simulink library "sm_mining_loader_lib"  (R2026a)
settings: Solver=VariableStepAuto
undefined symbols (not defined in the file): FL, FR, Init, LL, LR, Maneuver, minMachParams, motGradParams, RL, RR, simscape, SL, SR, T, X, Y, Z
libraries: sm_lib x130, nesl_utility x77, fl_lib x36, sdl_lib x11, simulink x4, $bdroot x3, sm_vehicle_utilities_lib x2, simulink_extras x2, statsLibrary x1, grid_element x1, Maneuver_Get_Pose x1
(part 1 of 6)
settings Model: Creator=smiller  LastModifiedBy=smiller

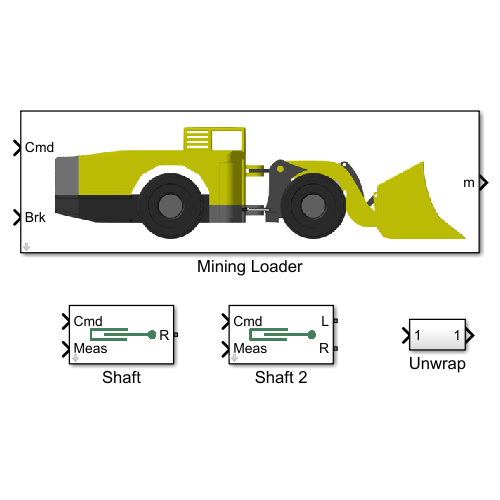
[thumbnail: Simulink's stored preview of the top-level diagram]
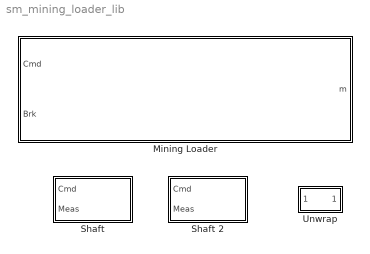
== system sm_mining_loader_lib ==
  Mining Loader : Subsystem  mask{popup_steer_actuation=Hinge Motion, popup_lift_actuation=Hinge Motion, popup_tilt_actuation=Hinge Motion, popup_scene=Grid, popup_sensor=None}
      mask prompts: popup_steer_actuation "Steer Actuation"; popup_lift_actuation "Lift Actuation"; popup_tilt_actuation "Tilt Actuation"; popup_scene "Scene"; popup_sensor "Sensor"
      mask init:
      | bh = gcb;
      | 
      | liftAct = get_param(bh,'popup_lift_actuation');
      | tiltAct = get_param(bh,'popup_tilt_actuation');
      | steerAct = get_param(bh,'popup_steer_actuation');
      | 
      | if(strcmp(liftAct,'Cylinder Actuation'))
      |     liftActStr = 'Shaft';
      | else
      |     liftActStr = 'Position';
      | end
      | if(strcmp(tiltAct,'Cylinder Actuation'))
      |     tiltActStr = 'Shaft';
      | else
      |     tiltActStr = 'Position';
      | end
      | if(strcmp(steerAct,'Cylinder Actuation'))
      |     steerActStr = 'Shaft';
      | else
      |     steerActStr = 'Position';
      | end
      | 
      | set_param([bh '/Actuation'],...
      |     'popup_lift_actuation',liftActStr,...
      |     'popup_tilt_actuation',tiltActStr,...
      |     'popup_steer_actuation',steerActStr...
      |     );
      | 
      | set_param([bh '/Scene'],...
      |     'LabelModeActiveChoice',get_param(bh,'popup_scene'))
      mask TypeOptions popup_steer_actuation: Vehicle/popup_steer_actuation
      mask TypeOptions popup_lift_actuation: Vehicle/popup_lift_actuation
      mask TypeOptions popup_tilt_actuation: Vehicle/popup_tilt_actuation
      mask TypeOptions popup_scene: SlopeX | Grid
      mask TypeOptions popup_sensor: Braking Distance Sensor/popup_sensor
      mask Display: image('sm_mining_loader_IMAGE.png')
  Shaft : Subsystem  VariantControl=Shaft  mask{Kp=motGradParams.bladeTilt.propGain, Ki=motGradParams.bladeTilt.integral, Kd=motGradParams.bladeTilt.derivative, p_init=motGradParams.bladeTilt.initPos, f_init=-4.07e4*3}
      mask prompts: Kp "Proportional Gain"; Ki "Integral Gain"; Kd "Derivative Gain"; p_init "Initial Position"; f_init "Initial Force"
      mask Display: image('sm_mining_loader_actuation_Shaft_IMAGE.png')
  Shaft 2 : Subsystem  VariantControl=Shaft  mask{Kp=minMachParams.Control.Steer.propGain, Ki=minMachParams.Control.Steer.intgGain, Kd=minMachParams.Control.Steer.dervGain, p_init=minMachParams.Control.Steer.initPos, popup_act_pair=Parallel}
      mask prompts: Kp "Proportional Gain"; Ki "Integral Gain"; Kd "Derivative Gain"; p_init "Initial Position"; popup_act_pair "Actuator Pair"
      mask init:
      | bh = gcb;
      | pairMode = get_param(bh,'popup_act_pair');
      | if(strcmp(pairMode,'Parallel'))
      | set_param([bh '/Sign L'],'Gain','1')
      | else
      |     set_param([bh '/Sign L'],'Gain','-1')
      | end
      mask TypeOptions popup_act_pair: Parallel | Opposing
      mask Display: image('sm_mining_loader_actuation_Shaft_IMAGE.png');
  Unwrap : Subsystem

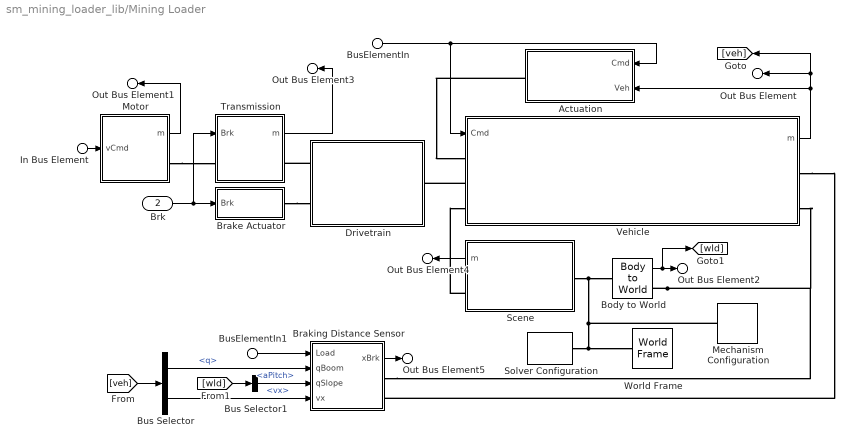
== system sm_mining_loader_lib/Mining Loader ==
  BusElementIn : Inport  PortName=Cmd
  In Bus Element : Inport  PortName=Cmd  Element=vVeh
  BusElementIn1 : Inport  PortName=Cmd  Element=Load
  Brk : Inport  Port=2
  Actuation : Subsystem  VariantControl=Actuation  mask{popup_steer_actuation=Position, popup_lift_actuation=Position, popup_tilt_actuation=Position}
      mask prompts: popup_steer_actuation "Steer Actuation"; popup_lift_actuation "Lift Actuation"; popup_tilt_actuation "Tilt Actuation"
      mask init:
      | bh = gcb;
      | 
      | set_param([bh '/Steer'],'LabelModeActiveChoice',get_param(bh,'popup_steer_actuation'))
      | set_param([bh '/Lift'],'LabelModeActiveChoice',get_param(bh,'popup_lift_actuation'))
      | set_param([bh '/Tilt'],'LabelModeActiveChoice',get_param(bh,'popup_tilt_actuation'))
      mask TypeOptions popup_steer_actuation: Position | Shaft
      mask TypeOptions popup_lift_actuation: Position | Shaft
      mask TypeOptions popup_tilt_actuation: Position | Shaft
  Body to World : sm_vehicle_utilities_lib/Body to World  Init=Init.Vehicle  SpecifyPosTarget=on
  Brake Actuator : Subsystem
  Braking Distance Sensor : Subsystem  Variant=on  VariantControlMode=label  LabelModeActiveChoice=None  mask{popup_sensor=None}
      mask prompts: popup_sensor "Sensor"
      mask init:
      | bh = gcb;
      | senseType = get_param(bh,'popup_sensor');
      | set_param(bh,'LabelModeActiveChoice',senseType);
      settings: AttributesFormatString=%<popup_sensor>
      mask TypeOptions popup_sensor: None | Estimate
      mask Display: disp(' ')
  Bus Selector : BusSelector  OutputSignals=Lift.H.q,Frame.Body.vx
  Bus Selector1 : BusSelector  OutputSignals=aPitch
  Drivetrain : Subsystem
      mask Display: image('sm_mining_loader_driveline_IMAGE.png');
  Mechanism Configuration : sm_lib/Utilities/Mechanism Configuration  UniformGravity=Constant  GravityVector=[0 0 -9.80665]  GravityVectorUnits=m/s^2  LinearizationDelta=0.001  JointModeTransitionNonlinearIterations=2
  Motor : Subsystem
      mask Display: image('sm_mining_loader_motor_ideal_IMAGE.png')
  Scene : Subsystem  Variant=on  VariantControlMode=label  LabelModeActiveChoice=Grid
  Solver Configuration : nesl_utility/Solver Configuration  PhysicalDomain=network_engine_domain  SubClassName=solver  LeftPortType=input  RightPortType=generic  Tones=[]  Harmonics=[]  SimulateNoise=off  Profile=off  UseLocalSampling=off  EnableSwitchedLinearOptims=on  FrequencyDomain=off  UseCCode=off  RelTol=0.001  AbsTol=0.001  MinStep=1e-09  ToWorkspace=off  RevertToSquareIcSolve=off  NumHomotopyIterations=100  PhasorMode=off  PhasorModeNumHarmonics=1  ConsistencySolver=NEWTON_XTOL_AFTER_FTOL  CanonicalOrdering=UNORDERED  OptimizeIntermediates=UNOPTIMIZED  IndexReductionMethod=DerivativeReplacement  DoDC=off  ResidualTolerance=1e-09  ConsistencyTolSource=GLOBAL  ConsistencyAbsTol=0.001  ConsistencyRelTol=0.001  ConsistencyTolFactor=0.001  UseLocalSolver=off  LocalSolverChoice=NE_BACKWARD_EULER_ADVANCER  ResolveIndetEquations=on  FunctionEvalNumThread=1  LocalSolverSampleTime=0.001  DoFixedCost=off  MaxNonlinIter=3  MaxModeIter=2  ComputeImpulses=off  ImpulseIterations=2  LinearAlgebra=auto  LinearAlgebraNumThread=0  EquationFormulation=NE_TIME_EF  DelaysMemoryBudget=1024  AutomaticFiltering=on  FilteringTimeConstant=0.001  PartitionStorageMethod=AS_NEEDED  PartitionMemoryBudget=1024  PartitionMethod=ROBUST  MultibodyUseLocalSolver=off  MultibodyLocalSolverChoice=ODE1  MultibodyLocalSolverSampleTime=0.001
  Transmission : Subsystem
      mask Display: image('sm_mining_loader_trans_IMAGE.png');
  Vehicle : Subsystem  mask{popup_steer_actuation=Hinge Motion, popup_lift_actuation=Hinge Motion, popup_tilt_actuation=Hinge Motion}
      mask prompts: popup_steer_actuation "Steer Actuation"; popup_lift_actuation "Lift Actuation"; popup_tilt_actuation "Tilt Actuation"
      mask TypeOptions popup_steer_actuation: Steer/popup_steer_actuation
      mask TypeOptions popup_lift_actuation: Implement/popup_lift_actuation
      mask TypeOptions popup_tilt_actuation: Implement/popup_tilt_actuation
      mask Display: image('sm_mining_loader_IMAGE.png')
  World Frame : sm_lib/Frames and Transforms/World Frame
  Out Bus Element : Outport  PortName=m  Element=Vehicle
  Out Bus Element1 : Outport  PortName=m  Element=Motor
  Out Bus Element2 : Outport  PortName=m  Element=World
  Out Bus Element3 : Outport  PortName=m  Element=Trans
  Out Bus Element4 : Outport  PortName=m  Element=Scene
  Out Bus Element5 : Outport  PortName=m  Element=Sensor.xBrk
  wires:
  Bus Selector1/1 -> Braking Distance Sensor/3(qSlope)  "<aPitch>"
  [wld] -> Bus Selector1/1
  Bus Selector/2 -> Braking Distance Sensor/4(vx)  "<vx>"
  Bus Selector/1 -> Braking Distance Sensor/2(qBoom)  "<q>"
  [veh] -> Bus Selector/1
  BusElementIn1/1 -> Braking Distance Sensor/1(Load)
  Vehicle/1(m) -> [veh], Out Bus Element/1, Actuation/2(Veh)
  BusElementIn/1 -> Vehicle/1(Cmd), Actuation/1(Cmd)
  Motor/1(m) -> Out Bus Element1/1
  Body to World/1 -> Out Bus Element2/1, [wld]
  Transmission/1(m) -> Out Bus Element3/1
  In Bus Element/1 -> Motor/1(vCmd)
  Brk/1 -> Brake Actuator/1(Brk), Transmission/1(Brk)
  Scene/1(m) -> Out Bus Element4/1
  Braking Distance Sensor/1(xBrk) -> Out Bus Element5/1
  connections:
  Scene/LConn1 -- Body to World/LConn1 -- Mechanism Configuration/RConn1 -- Solver Configuration/RConn1 -- World Frame/RConn1
  Brake Actuator/RConn1 -- Drivetrain/LConn2
  Body to World/RConn1 -- Vehicle/RConn2 -- Braking Distance Sensor/RConn1
  Vehicle/LConn2 -- Drivetrain/RConn1
  Actuation/RConn1 -- Vehicle/LConn1
  Scene/RConn1 -- Vehicle/LConn3
  Motor/RConn1 -- Transmission/LConn1
  Drivetrain/LConn1 -- Transmission/RConn1
  Vehicle/RConn1 -- Braking Distance Sensor/RConn2

== system sm_mining_loader_lib/Shaft ==
  Cmd : Inport
  Meas : Inport  Port=2
  Force Source : fl_lib/Mechanical/Mechanical Sources/Ideal Force Source
  Gain : Gain  Gain=Kp
  Gain1 : Gain  Gain=Ki
  Gain2 : Gain  Gain=Kd
  Integrator : Integrator  InitialCondition=f_init
  Mechanical Translational Reference2 : fl_lib/Mechanical/Translational Elements/Mechanical Translational Reference
  Simulink-PS Converter2 : nesl_utility/Simulink-PS Converter  PhysicalDomain=network_engine_domain  SubClassName=ps_input  LeftPortType=input  RightPortType=output  PseudoPeriodic=off  Frequencies=[]  NoiseDistribution=none  NoiseParameters=[]  Unit=1  AffineConversion=off  FilteringAndDerivatives=provide  SimscapeFilterOrder=1  InputFilterTimeConstant=0.001  UdotUserProvided=0
  Subtract : Sum  Inputs=+-
  Sum1 : Sum  Inputs=+++
  Transfer Fcn : TransferFcn  Numerator=[1 0]  Denominator=[0.01 1]
  Transfer Fcn (with initial outputs) : simulink_extras/Additional Linear/Transfer Fcn (with initial outputs)  N=[1]  D="[0.01  1]"  Y0=p_init  U0=p_init
  R : PMIOPort  Side=Right
  wires:
  Integrator/1 -> Sum1/2
  Gain/1 -> Sum1/1
  Transfer Fcn (with initial outputs)/1 -> Subtract/2
  Sum1/1 -> Simulink-PS Converter2/1  "Force Command"
  Meas/1 -> Transfer Fcn (with initial outputs)/1
  Cmd/1 -> Subtract/1
  Gain1/1 -> Integrator/1
  Gain2/1 -> Transfer Fcn/1
  Subtract/1 -> Gain2/1, Gain1/1, Gain/1
  Transfer Fcn/1 -> Sum1/3
  connections:
  Force Source/RConn2 -- Mechanical Translational Reference2/LConn1
  Simulink-PS Converter2/RConn1 -- Force Source/RConn1
  R/RConn1 -- Force Source/LConn1

== system sm_mining_loader_lib/Shaft 2 ==
  Cmd : Inport
  Meas : Inport  Port=2
  Force Source L : fl_lib/Mechanical/Mechanical Sources/Ideal Force Source
  Force Source R : fl_lib/Mechanical/Mechanical Sources/Ideal Force Source
  Gain : Gain  Gain=Kp
  Gain1 : Gain  Gain=Ki
  Gain2 : Gain  Gain=Kd
  Integrator : Integrator
  Mechanical Translational Reference1 : fl_lib/Mechanical/Translational Elements/Mechanical Translational Reference
  Mechanical Translational Reference2 : fl_lib/Mechanical/Translational Elements/Mechanical Translational Reference
  Sign L : Gain
  Sign R : Gain
  Simulink-PS Converter1 : nesl_utility/Simulink-PS Converter  PhysicalDomain=network_engine_domain  SubClassName=ps_input  LeftPortType=input  RightPortType=output  PseudoPeriodic=off  Frequencies=[]  NoiseDistribution=none  NoiseParameters=[]  Unit=1  AffineConversion=off  FilteringAndDerivatives=provide  SimscapeFilterOrder=1  InputFilterTimeConstant=0.001  UdotUserProvided=0
  Simulink-PS Converter2 : nesl_utility/Simulink-PS Converter  PhysicalDomain=network_engine_domain  SubClassName=ps_input  LeftPortType=input  RightPortType=output  PseudoPeriodic=off  Frequencies=[]  NoiseDistribution=none  NoiseParameters=[]  Unit=1  AffineConversion=off  FilteringAndDerivatives=provide  SimscapeFilterOrder=1  InputFilterTimeConstant=0.001  UdotUserProvided=0
  Subtract : Sum  Inputs=+-
  Sum1 : Sum  Inputs=+++
  Transfer Fcn : TransferFcn  Numerator=[1 0]  Denominator=[0.01 1]
  Transfer Fcn (with initial outputs) : simulink_extras/Additional Linear/Transfer Fcn (with initial outputs)  N=[1]  D="[0.01  1]"  Y0=p_init  U0=p_init
  L : PMIOPort  Side=Right
  R : PMIOPort  Port=2  Side=Right
  wires:
  Transfer Fcn/1 -> Sum1/3
  Subtract/1 -> Gain/1, Gain1/1, Gain2/1
  Gain2/1 -> Transfer Fcn/1
  Gain1/1 -> Integrator/1
  Cmd/1 -> Subtract/1
  Sum1/1 -> Sign L/1, Sign R/1  "Force Command"
  Transfer Fcn (with initial outputs)/1 -> Subtract/2
  Gain/1 -> Sum1/1
  Integrator/1 -> Sum1/2
  Sign R/1 -> Simulink-PS Converter1/1
  Sign L/1 -> Simulink-PS Converter2/1
  Meas/1 -> Transfer Fcn (with initial outputs)/1
  connections:
  L/RConn1 -- Force Source L/LConn1
  Simulink-PS Converter2/RConn1 -- Force Source L/RConn1
  Force Source L/RConn2 -- Mechanical Translational Reference2/LConn1
  Force Source R/RConn2 -- Mechanical Translational Reference1/LConn1
  Simulink-PS Converter1/RConn1 -- Force Source R/RConn1
  R/RConn1 -- Force Source R/LConn1

== system sm_mining_loader_lib/Unwrap ==
  In1 : Inport
  Compare To Constant : simulink/Logic and Bit Operations/Compare To Constant  relop=>  const=pi  OutDataTypeStr=boolean
  Compare To Constant1 : simulink/Logic and Bit Operations/Compare To Constant  relop=<  const=-pi  OutDataTypeStr=boolean
  Data Type Conversion : DataTypeConversion  SaturateOnIntegerOverflow=off  RndMeth=Floor
  Data Type Conversion1 : DataTypeConversion  SaturateOnIntegerOverflow=off  RndMeth=Floor
  Gain5 : Gain  Gain=2*pi
  Memory : Memory
  OR : Logic  Operator=OR  IconShape=distinctive  AllPortsSameDT=off  OutDataTypeStr=boolean
  Scope : Scope  NumInputPorts=2
      settings: ActiveDisplayYMinimum=-4.3196898986858123  ActiveDisplayYMaximum=7.4612825522752164  DataLoggingVariableName=ScopeData8
  Subtract1 : Sum  Inputs=+-
  Sum : Sum  Inputs=+-|
  Sum2 : Sum  Inputs=|++
  Triggered Subsystem : Maneuver_Get_Pose/Maneuver/PoseTargetVisual/Count Lap/Triggered Subsystem  SystemSampleTime=-1  VariantActivationTime=update diagram  EmptyChoice=off  PassThrough=off  PassThroughVariantControl=(default)  EmptyChoiceVariantControl=(default)  AllowFlexibleInterface=on  Latency=0  AutoFrameSizeCalculation=off
  Out1 : Outport
  wires:
  Sum2/1 -> Out1/1
  Sum/1 -> Triggered Subsystem/1  "Counter"
  Data Type Conversion1/1 -> Sum/2
  OR/1 -> Triggered Subsystem/Trigger  "Trigger"
  Gain5/1 -> Sum2/2
  Memory/1 -> Subtract1/2
  Data Type Conversion/1 -> Sum/1
  Compare To Constant/1 -> Data Type Conversion1/1, OR/2  "Subtract Lap"
  In1/1 -> Scope/1, Subtract1/1, Memory/1, Sum2/1
  Compare To Constant1/1 -> Data Type Conversion/1, OR/1  "Add Lap"
  Subtract1/1 -> Scope/2, Compare To Constant1/1, Compare To Constant/1
  Triggered Subsystem/1 -> Gain5/1

== system sm_mining_loader_lib/Mining Loader/Actuation ==
  BusElementIn : Inport  PortName=Cmd  Element=qStr
  BusElementIn1 : Inport  PortName=Cmd  Element=qBoom
  BusElementIn2 : Inport  PortName=Cmd  Element=qBucket
  BusElementIn4 : Inport  Port=2  PortName=Veh  Element=Steer.H.q
  BusElementIn5 : Inport  Port=2  PortName=Veh  Element=Tilt.H.q
  BusElementIn6 : Inport  Port=2  PortName=Veh  Element=Lift.H.q
  Lift : Subsystem  Variant=on  VariantControlMode=label  LabelModeActiveChoice=Position
  Simscape Bus1 : SimscapeBus  HierarchyStrings=SL;SR;LL;LR;T
  Steer : Subsystem  Variant=on  VariantControlMode=label  LabelModeActiveChoice=Position
  Tilt : Subsystem  Variant=on  VariantControlMode=label  LabelModeActiveChoice=Position
  Act : PMIOPort  Side=Right
  wires:
  BusElementIn/1 -> Steer/1(Cmd)
  BusElementIn1/1 -> Lift/1(Cmd)
  BusElementIn2/1 -> Tilt/1(Cmd)
  BusElementIn4/1 -> Steer/2(Meas)
  BusElementIn6/1 -> Lift/2(Meas)
  BusElementIn5/1 -> Tilt/2(Meas)
  connections:
  Simscape Bus1/RConn1 -- Act/RConn1
  Steer/RConn1 -- Simscape Bus1/LConn1
  Steer/RConn2 -- Simscape Bus1/LConn2
  Lift/RConn1 -- Simscape Bus1/LConn3
  Lift/RConn2 -- Simscape Bus1/LConn4
  Tilt/RConn1 -- Simscape Bus1/LConn5

== system sm_mining_loader_lib/Mining Loader/Brake Actuator ==
  Brk : Inport
  LowHydraulicPressure : fl_lib/Physical Signals/Sources/PS Constant  constant=1e2 Pa
  MaxHydraulicPressure : fl_lib/Physical Signals/Sources/PS Constant  constant=minMachParams.braking.maxHydraulicPres Pa
  PS Switch : fl_lib/Physical Signals/Nonlinear Operators/PS Switch  Threshold=1  ZeroCross=true
  PS Transfer Function : fl_lib/Physical Signals/Linear Operators/PS Transfer Function  transfer_function_type=foundation.enum.transfer_function_type.lag  T=0.01 s  T1=2 s  T2=1 s  reset_method=foundation.enum.IntegratorResetSpec.None  initial_condition_spec=foundation.enum.IntegratorICSpec.Internal  y0=minMachParams.braking.maxHydraulicPres Pa
  Simulink-PS Converter3 : nesl_utility/Simulink-PS Converter  PhysicalDomain=network_engine_domain  SubClassName=ps_input  LeftPortType=input  RightPortType=output  PseudoPeriodic=off  Frequencies=[]  NoiseDistribution=none  NoiseParameters=[]  Unit=1  AffineConversion=off  FilteringAndDerivatives=provide  SimscapeFilterOrder=1  InputFilterTimeConstant=0.001  UdotUserProvided=0
  pBrk : PMIOPort  Side=Right
  wires:
  Brk/1 -> Simulink-PS Converter3/1
  connections:
  Simulink-PS Converter3/RConn1 -- PS Switch/LConn2
  MaxHydraulicPressure/RConn1 -- PS Switch/LConn1
  LowHydraulicPressure/RConn1 -- PS Switch/LConn3
  PS Switch/RConn1 -- PS Transfer Function/LConn1
  PS Transfer Function/RConn1 -- pBrk/RConn1

== system sm_mining_loader_lib/Mining Loader/Braking Distance Sensor ==
  Load : Inport
  qBoom : Inport  Port=2
  qSlope : Inport  Port=3
  vx : Inport  Port=4
  Estimate : Subsystem  VariantControl=Estimate  mask{TsVis=minMachParams.visual.Ts}
      mask prompts: TsVis "Sample Time (s)"
      mask TypeOptions TsVis: Unit Delay/SampleTime | Unit Delay1/SampleTime
  None : Subsystem  VariantControl=None
  RefF : PMIOPort  Side=Right
  RefR : PMIOPort  Port=2  Side=Right
  xBrk : Outport

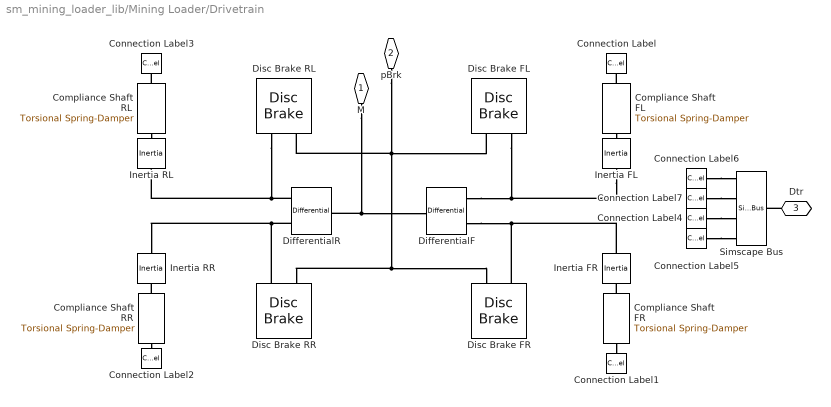
== system sm_mining_loader_lib/Mining Loader/Drivetrain ==
  Compliance Shaft FL : sdl_lib/Couplings & Drives/Torsional Spring-Damper  k=minMachParams.driveshaft.k N*m/rad  mu_visc=minMachParams.driveshaft.d N*m*s/rad  trq_coulomb=minMachParams.driveshaft.trqCou N*m  static_kinetic_ratio=minMachParams.driveshaft.sta2Kin  w_tol=minMachParams.driveshaft.wTol rad/s  model_hardstop=sdl.enum.hardStopOffOn.off  upper_bound=10 deg  lower_bound=-10 deg  hardstop_model=simscape.enum.hardstop.smooth  k_endstop=1e6 N*m/rad  D_endstop=10 N*m*s/rad  transition=0.001 rad  coeff_rest=0.7  w_tol_hardstop=0.1 rad/s  trq_tol=0.001 N*m  x0=0 deg
  Compliance Shaft FR : sdl_lib/Couplings & Drives/Torsional Spring-Damper  k=minMachParams.driveshaft.k N*m/rad  mu_visc=minMachParams.driveshaft.d N*m*s/rad  trq_coulomb=minMachParams.driveshaft.trqCou N*m  static_kinetic_ratio=minMachParams.driveshaft.sta2Kin  w_tol=minMachParams.driveshaft.wTol rad/s  model_hardstop=sdl.enum.hardStopOffOn.off  upper_bound=10 deg  lower_bound=-10 deg  hardstop_model=simscape.enum.hardstop.smooth  k_endstop=1e6 N*m/rad  D_endstop=10 N*m*s/rad  transition=0.001 rad  coeff_rest=0.7  w_tol_hardstop=0.1 rad/s  trq_tol=0.001 N*m  x0=0 deg
  Compliance Shaft RL : sdl_lib/Couplings & Drives/Torsional Spring-Damper  k=minMachParams.driveshaft.k N*m/rad  mu_visc=minMachParams.driveshaft.d N*m*s/rad  trq_coulomb=minMachParams.driveshaft.trqCou N*m  static_kinetic_ratio=minMachParams.driveshaft.sta2Kin  w_tol=minMachParams.driveshaft.wTol rad/s  model_hardstop=sdl.enum.hardStopOffOn.off  upper_bound=10 deg  lower_bound=-10 deg  hardstop_model=simscape.enum.hardstop.smooth  k_endstop=1e6 N*m/rad  D_endstop=10 N*m*s/rad  transition=0.001 rad  coeff_rest=0.7  w_tol_hardstop=0.1 rad/s  trq_tol=0.001 N*m  x0=0 deg
  Compliance Shaft RR : sdl_lib/Couplings & Drives/Torsional Spring-Damper  k=minMachParams.driveshaft.k N*m/rad  mu_visc=minMachParams.driveshaft.d N*m*s/rad  trq_coulomb=minMachParams.driveshaft.trqCou N*m  static_kinetic_ratio=minMachParams.driveshaft.sta2Kin  w_tol=minMachParams.driveshaft.wTol rad/s  model_hardstop=sdl.enum.hardStopOffOn.off  upper_bound=10 deg  lower_bound=-10 deg  hardstop_model=simscape.enum.hardstop.smooth  k_endstop=1e6 N*m/rad  D_endstop=10 N*m*s/rad  transition=0.001 rad  coeff_rest=0.7  w_tol_hardstop=0.1 rad/s  trq_tol=0.001 N*m  x0=0 deg
  Connection Label : ConnectionLabel  Label=FL
  Connection Label1 : ConnectionLabel  Label=FR
  Connection Label2 : ConnectionLabel  Label=RR
  Connection Label3 : ConnectionLabel  Label=RL
  Connection Label4 : ConnectionLabel  Label=FR
  Connection Label5 : ConnectionLabel  Label=FL
  Connection Label6 : ConnectionLabel  Label=RR
  Connection Label7 : ConnectionLabel  Label=RL
  DifferentialF : sdl_lib/Gears/Differential  driveshaft_location=sdl.enum.differential_orientation.left  cd_ratio=1  friction_model=sdl.enum.gear_friction.none  efficiency=[.85, .92]  temperature_TLU=[280, 300, 320] K  efficiency_ss_TLU=[.95, .9, .85]  efficiency_cd_TLU=[.95, .9, .85]  pwr_thr=[.001, .001] W  mu_visc=[0, 0] N*m*s/rad  model_inertia=simscape.enum.onoff.off  sun_inertia=0.001 kg*m^2  sun_radius=0.01 m  carrier_inertia=0.001 kg*m^2  planet_inertia=0.001 kg*m^2  planet_mass=0.001 kg  thermal_mass=50 J/K  T_init=300 K
  DifferentialR : sdl_lib/Gears/Differential  driveshaft_location=sdl.enum.differential_orientation.left  cd_ratio=1  friction_model=sdl.enum.gear_friction.none  efficiency=[.85, .92]  temperature_TLU=[280, 300, 320] K  efficiency_ss_TLU=[.95, .9, .85]  efficiency_cd_TLU=[.95, .9, .85]  pwr_thr=[.001, .001] W  mu_visc=[0, 0] N*m*s/rad  model_inertia=simscape.enum.onoff.off  sun_inertia=0.001 kg*m^2  sun_radius=0.01 m  carrier_inertia=0.001 kg*m^2  planet_inertia=0.001 kg*m^2  planet_mass=0.001 kg  thermal_mass=50 J/K  T_init=300 K
  Disc Brake FL : sdl_lib/Brakes & Detents/Rotational/Disc Brake  r_mean=minMachParams.braking.meanPadRadius mm  bore=minMachParams.braking.cylinderBore m  n_pads=minMachParams.braking.numPads  thermal_port=simscape.enum.thermaleffects.omit  mu_static=minMachParams.braking.staticFriction  mu_coulomb=minMachParams.braking.kineticFriction  temperature_TLU=[280, 300, 320] K  mu_static_TLU=[.9, .8, .7]  mu_coulomb_TLU=[.8, .7, .6]  brkwy_vel=minMachParams.braking.breakawayFricVel rad/s  visc_coef=minMachParams.braking.viscousFricCoeff N*m*s/rad  thermal_mass=50 kJ/K  temperature_specify=off  temperature_priority=High  temperature=300 K  temperature_nominal_specify=off  temperature_nominal_value=1  temperature_nominal_unit=K
  Disc Brake FR : sdl_lib/Brakes & Detents/Rotational/Disc Brake  r_mean=minMachParams.braking.meanPadRadius mm  bore=minMachParams.braking.cylinderBore m  n_pads=minMachParams.braking.numPads  thermal_port=simscape.enum.thermaleffects.omit  mu_static=minMachParams.braking.staticFriction  mu_coulomb=minMachParams.braking.kineticFriction  temperature_TLU=[280, 300, 320] K  mu_static_TLU=[.9, .8, .7]  mu_coulomb_TLU=[.8, .7, .6]  brkwy_vel=minMachParams.braking.breakawayFricVel rad/s  visc_coef=minMachParams.braking.viscousFricCoeff N*m*s/rad  thermal_mass=50 kJ/K  temperature_specify=off  temperature_priority=High  temperature=300 K  temperature_nominal_specify=off  temperature_nominal_value=1  temperature_nominal_unit=K
  Disc Brake RL : sdl_lib/Brakes & Detents/Rotational/Disc Brake  r_mean=minMachParams.braking.meanPadRadius mm  bore=minMachParams.braking.cylinderBore m  n_pads=minMachParams.braking.numPads  thermal_port=simscape.enum.thermaleffects.omit  mu_static=minMachParams.braking.staticFriction  mu_coulomb=minMachParams.braking.kineticFriction  temperature_TLU=[280, 300, 320] K  mu_static_TLU=[.9, .8, .7]  mu_coulomb_TLU=[.8, .7, .6]  brkwy_vel=minMachParams.braking.breakawayFricVel rad/s  visc_coef=minMachParams.braking.viscousFricCoeff N*m*s/rad  thermal_mass=50 kJ/K  temperature_specify=off  temperature_priority=High  temperature=300 K  temperature_nominal_specify=off  temperature_nominal_value=1  temperature_nominal_unit=K
  Disc Brake RR : sdl_lib/Brakes & Detents/Rotational/Disc Brake  r_mean=minMachParams.braking.meanPadRadius mm  bore=minMachParams.braking.cylinderBore m  n_pads=minMachParams.braking.numPads  thermal_port=simscape.enum.thermaleffects.omit  mu_static=minMachParams.braking.staticFriction  mu_coulomb=minMachParams.braking.kineticFriction  temperature_TLU=[280, 300, 320] K  mu_static_TLU=[.9, .8, .7]  mu_coulomb_TLU=[.8, .7, .6]  brkwy_vel=minMachParams.braking.breakawayFricVel rad/s  visc_coef=minMachParams.braking.viscousFricCoeff N*m*s/rad  thermal_mass=50 kJ/K  temperature_specify=off  temperature_priority=High  temperature=300 K  temperature_nominal_specify=off  temperature_nominal_value=1  temperature_nominal_unit=K
  Inertia FL : fl_lib/Mechanical/Rotational Elements/Inertia  inertia=minMachParams.driveshaft.J kg*m^2  num_ports=foundation.enum.numPorts2.two  w_specify=off  w_priority=High  w=0 rad/s  w_nominal_specify=off  w_nominal_value=1  w_nominal_unit=rad/s  t_specify=off  t_priority=None  t=0 N*m  t_nominal_specify=off  t_nominal_value=1  t_nominal_unit=N*m
  Inertia FR : fl_lib/Mechanical/Rotational Elements/Inertia  inertia=minMachParams.driveshaft.J kg*m^2  num_ports=foundation.enum.numPorts2.two  w_specify=off  w_priority=High  w=0 rad/s  w_nominal_specify=off  w_nominal_value=1  w_nominal_unit=rad/s  t_specify=off  t_priority=None  t=0 N*m  t_nominal_specify=off  t_nominal_value=1  t_nominal_unit=N*m
  Inertia RL : fl_lib/Mechanical/Rotational Elements/Inertia  inertia=minMachParams.driveshaft.J kg*m^2  num_ports=foundation.enum.numPorts2.two  w_specify=off  w_priority=High  w=0 rad/s  w_nominal_specify=off  w_nominal_value=1  w_nominal_unit=rad/s  t_specify=off  t_priority=None  t=0 N*m  t_nominal_specify=off  t_nominal_value=1  t_nominal_unit=N*m
  Inertia RR : fl_lib/Mechanical/Rotational Elements/Inertia  inertia=minMachParams.driveshaft.J kg*m^2  num_ports=foundation.enum.numPorts2.two  w_specify=off  w_priority=High  w=0 rad/s  w_nominal_specify=off  w_nominal_value=1  w_nominal_unit=rad/s  t_specify=off  t_priority=None  t=0 N*m  t_nominal_specify=off  t_nominal_value=1  t_nominal_unit=N*m
  Simscape Bus : SimscapeBus  HierarchyStrings=RR;RL;FR;FL
  M : PMIOPort  Side=Left
  pBrk : PMIOPort  Port=2  Side=Left
  Dtr : PMIOPort  Port=3  Side=Right
  connections:
  Compliance Shaft RR/LConn1 -- Connection Label2/LConn1
  Compliance Shaft FL/LConn1 -- Connection Label/LConn1
  DifferentialR/RConn2 -- Inertia RL/LConn1 -- Disc Brake RL/LConn2
  pBrk/RConn1 -- Disc Brake FR/LConn1 -- Disc Brake RR/LConn1 -- Disc Brake FL/LConn1 -- Disc Brake RL/LConn1
  Compliance Shaft RL/LConn1 -- Connection Label3/LConn1
  DifferentialR/RConn1 -- Disc Brake RR/LConn2 -- Inertia RR/RConn1
  M/RConn1 -- DifferentialR/LConn1 -- DifferentialF/LConn1
  DifferentialF/RConn1 -- Inertia FR/RConn1 -- Disc Brake FR/LConn2
  DifferentialF/RConn2 -- Disc Brake FL/LConn2 -- Inertia FL/LConn1
  Connection Label4/LConn1 -- Simscape Bus/LConn3
  Connection Label5/LConn1 -- Simscape Bus/LConn4
  Connection Label6/LConn1 -- Simscape Bus/LConn1
  Connection Label7/LConn1 -- Simscape Bus/LConn2
  Dtr/RConn1 -- Simscape Bus/RConn1
  Compliance Shaft FR/LConn1 -- Connection Label1/LConn1
  Compliance Shaft RR/RConn1 -- Inertia RR/LConn1
  Compliance Shaft RL/RConn1 -- Inertia RL/RConn1
  Compliance Shaft FL/RConn1 -- Inertia FL/RConn1
  Compliance Shaft FR/RConn1 -- Inertia FR/LConn1

== system sm_mining_loader_lib/Mining Loader/Motor ==
  vCmd : Inport
  Constant : Constant  Value=minMachParams.contact.tireRad
  Divide : Product  Inputs=*/
  Gain : Gain  Gain=1e3/3600
  Gain1 : Gain  Gain=1/1000
  Ideal Angular Velocity Source : fl_lib/Mechanical/Mechanical Sources/Ideal Angular Velocity Source
  Ideal Torque Sensor : fl_lib/Mechanical/Mechanical Sensors/Ideal Torque Sensor
  Mechanical Rotational Reference1 : fl_lib/Mechanical/Rotational Elements/Mechanical Rotational Reference
  PS-Simulink Converter : nesl_utility/PS-Simulink Converter  PhysicalDomain=network_engine_domain  SubClassName=ps_output  LeftPortType=input  RightPortType=output  PseudoPeriodic=off  Frequencies=[]  VectorFormat=inherit  Unit=inherit  AffineConversion=off
  Simulink-PS Converter2 : nesl_utility/Simulink-PS Converter  PhysicalDomain=network_engine_domain  SubClassName=ps_input  LeftPortType=input  RightPortType=output  PseudoPeriodic=off  Frequencies=[]  NoiseDistribution=none  NoiseParameters=[]  Unit=rad/s  AffineConversion=off  FilteringAndDerivatives=filter  SimscapeFilterOrder=2  InputFilterTimeConstant=0.001  UdotUserProvided=0
  Transfer Fcn : TransferFcn  Denominator=[0.1 1]
  R : PMIOPort  Side=Right
  Out Bus Element : Outport  PortName=m  Element=trq
  wires:
  Transfer Fcn/1 -> Divide/1
  Gain/1 -> Transfer Fcn/1
  Gain1/1 -> Divide/2
  Constant/1 -> Gain1/1
  vCmd/1 -> Gain/1
  Divide/1 -> Simulink-PS Converter2/1
  PS-Simulink Converter/1 -> Out Bus Element/1
  connections:
  Simulink-PS Converter2/RConn1 -- Ideal Angular Velocity Source/RConn1
  Mechanical Rotational Reference1/LConn1 -- Ideal Angular Velocity Source/RConn2
  Ideal Angular Velocity Source/LConn1 -- Ideal Torque Sensor/RConn1
  R/RConn1 -- Ideal Torque Sensor/LConn1
  Ideal Torque Sensor/RConn2 -- PS-Simulink Converter/LConn1

== system sm_mining_loader_lib/Mining Loader/Scene ==
  Grid : Subsystem  VariantControl=Grid
      mask Display: image('sm_mining_loader_scene_grid_IMAGE.png')
  SlopeX : Subsystem  VariantControl=SlopeX
      mask Display: image('sm_mining_loader_scene_slopex_IMAGE.png');
  G : PMIOPort  Side=Right
  W : PMIOPort  Port=2  Side=Left
  m : Outport

== system sm_mining_loader_lib/Mining Loader/Transmission ==
  Brk : Inport
  Constant1 : Constant  Value=0
  Constant2 : Constant
  Ideal Rotational Motion Sensor : fl_lib/Mechanical/Mechanical Sensors/Ideal Rotational Motion Sensor  reference=foundation.enum.MeasurementReference.absolute  acceleration_port=false  velocity_port=true  position_port=false  wrap_angle=false  offset=0 rad
  PS-Simulink Converter : nesl_utility/PS-Simulink Converter  PhysicalDomain=network_engine_domain  SubClassName=ps_output  LeftPortType=input  RightPortType=output  PseudoPeriodic=off  Frequencies=[]  VectorFormat=inherit  Unit=inherit  AffineConversion=off
  Simulink-PS Converter3 : nesl_utility/Simulink-PS Converter  PhysicalDomain=network_engine_domain  SubClassName=ps_input  LeftPortType=input  RightPortType=output  PseudoPeriodic=off  Frequencies=[]  NoiseDistribution=none  NoiseParameters=[]  Unit=1  AffineConversion=off  FilteringAndDerivatives=provide  SimscapeFilterOrder=1  InputFilterTimeConstant=0.001  UdotUserProvided=0
  Switch : Switch  Criteria=u2 > Threshold  Threshold=0.5  SaturateOnIntegerOverflow=off  InputSameDT=off
  Variable Ratio Transmission : sdl_lib/Couplings & Drives/Variable Ratio Transmission  rotation_direction=sdl.enum.shaftOutputDirection.same  kp=1e7 N*m/rad  kv=5e6 N*m*s/rad  initial_torque=0 N*m  ratio_thr=0.01  losses_model=sdl.enum.lossesOffOn.off  efficiency=0.8  pwr_thr=0.001 W  mu_visc=[0, 0] N*m*s/rad
  F : PMIOPort  Side=Right
  B : PMIOPort  Port=2  Side=Left
  Out Bus Element : Outport  PortName=m  Element=wOut
  wires:
  Constant1/1 -> Switch/1
  Constant2/1 -> Switch/3
  Switch/1 -> Simulink-PS Converter3/1
  Brk/1 -> Switch/2
  PS-Simulink Converter/1 -> Out Bus Element/1
  connections:
  Ideal Rotational Motion Sensor/RConn1 -- PS-Simulink Converter/LConn1
  Simulink-PS Converter3/RConn1 -- Variable Ratio Transmission/LConn1
  Variable Ratio Transmission/RConn1 -- F/RConn1 -- Ideal Rotational Motion Sensor/LConn1
  B/RConn1 -- Variable Ratio Transmission/LConn2

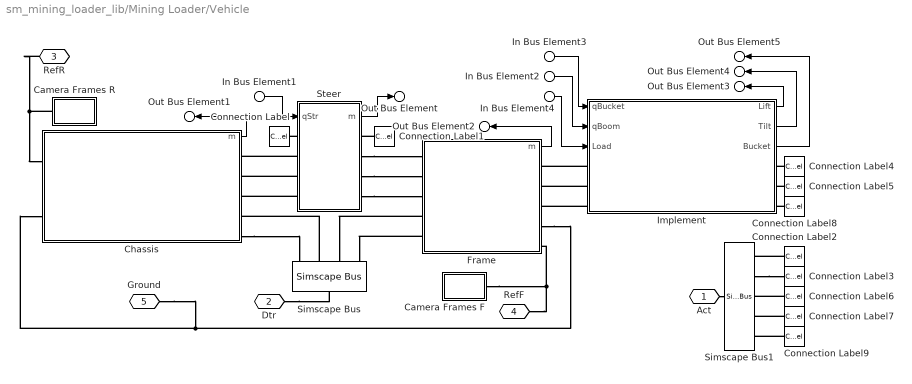
== system sm_mining_loader_lib/Mining Loader/Vehicle ==
  In Bus Element1 : Inport  PortName=Cmd  Element=qStr
  In Bus Element2 : Inport  PortName=Cmd  Element=qBoom
  In Bus Element3 : Inport  PortName=Cmd  Element=qBucket
  In Bus Element4 : Inport  PortName=Cmd  Element=Load
  Camera Frames F : Subsystem
  Camera Frames R : Subsystem
  Chassis : Subsystem
      mask Display: image('sm_mining_loader_chassis_IMAGE.png')
  Connection Label : ConnectionLabel  Label=SL
  Connection Label1 : ConnectionLabel  Label=SR
  Connection Label2 : ConnectionLabel  Label=SL
  Connection Label3 : ConnectionLabel  Label=SR
  Connection Label4 : ConnectionLabel  Label=LL
  Connection Label5 : ConnectionLabel  Label=LR
  Connection Label6 : ConnectionLabel  Label=LL
  Connection Label7 : ConnectionLabel  Label=LR
  Connection Label8 : ConnectionLabel  Label=T
  Connection Label9 : ConnectionLabel  Label=T
  Frame : Subsystem
      mask Display: image('sm_mining_loader_frame_IMAGE.png')
  Implement : Subsystem  mask{popup_lift_actuation=Hinge Motion, popup_tilt_actuation=Hinge Motion}
      mask prompts: popup_lift_actuation "Lift Actuation"; popup_tilt_actuation "Tilt Actuation"
      mask TypeOptions popup_lift_actuation: Lift Actuators/popup_lift_actuation
      mask TypeOptions popup_tilt_actuation: Tilt Actuator/popup_tilt_actuation
      mask Display: image('sm_mining_loader_impl_IMAGE.png')
  Simscape Bus : SimscapeBus  HierarchyStrings=RR;RL;FR;FL
  Simscape Bus1 : SimscapeBus  HierarchyStrings=SL;SR;LL;LR;T
  Steer : Subsystem  mask{popup_steer_actuation=Hinge Motion}
      mask prompts: popup_steer_actuation "Steer Actuation"
      mask init:
      | bh = gcb;
      | 
      | actSetting = get_param(bh,'popup_steer_actuation');
      | 
      | switch actSetting
      |     case('Hinge Motion')
      |         labelStr = 'Hinge';
      |     case('Left Cylinder Motion')
      |         labelStr = 'Extension_L';
      |     case('Cylinder Actuation')
      |         labelStr = 'Actuation';
      | end
      | set_param([bh '/Actuation'],'LabelModeActiveChoice',labelStr)
      settings: AttributesFormatString=%<popup_steer_actuation>
      mask TypeOptions popup_steer_actuation: Hinge Motion | Left Cylinder Motion | Cylinder Actuation
      mask Display:
      | bh = gcb;
      | 
      | actSetting = get_param(bh,'popup_steer_actuation');
      | 
      | switch actSetting
      |     case('Hinge Motion')
      |         imageStr = 'sm_mining_loader_steer_hinge_motion_IMAGE.png';
      |     case('Left Cylinder Motion')
      |         imageStr = 'sm_mining_loader_steer_cyl_motion_IMAGE.png';
      |     case('Cylinder Actuation')
      |         imageStr = 'sm_mining_loader_steer_cyl_actuation_IMAGE.png';
      | end
      | image(imageStr)
  Act : PMIOPort  Side=Left
  Dtr : PMIOPort  Port=2  Side=Left
  RefR : PMIOPort  Port=3  Side=Right
  RefF : PMIOPort  Port=4  Side=Right
  Ground : PMIOPort  Port=5  Side=Left
  Out Bus Element : Outport  PortName=m  Element=Steer
  Out Bus Element1 : Outport  PortName=m  Element=Chassis
  Out Bus Element2 : Outport  PortName=m  Element=Frame
  Out Bus Element3 : Outport  PortName=m  Element=Lift
  Out Bus Element4 : Outport  PortName=m  Element=Tilt
  Out Bus Element5 : Outport  PortName=m  Element=Bucket
  wires:
  In Bus Element3/1 -> Implement/1(qBucket)
  In Bus Element2/1 -> Implement/2(qBoom)
  Steer/1(m) -> Out Bus Element/1
  Chassis/1(m) -> Out Bus Element1/1
  Frame/1(m) -> Out Bus Element2/1
  Implement/1(Lift) -> Out Bus Element3/1
  Implement/2(Tilt) -> Out Bus Element4/1
  In Bus Element1/1 -> Steer/1(qStr)
  Implement/3(Bucket) -> Out Bus Element5/1
  In Bus Element4/1 -> Implement/3(Load)
  connections:
  Frame/RConn4 -- Ground/RConn1 -- Chassis/LConn2
  Implement/LConn3 -- Frame/RConn3
  Implement/LConn1 -- Frame/RConn1
  Implement/LConn2 -- Frame/RConn2
  Frame/LConn4 -- Simscape Bus/LConn3
  Frame/LConn5 -- Simscape Bus/LConn4
  Steer/LConn2 -- Chassis/RConn1
  Steer/LConn3 -- Chassis/RConn2
  Steer/RConn2 -- Frame/LConn1
  Steer/RConn3 -- Frame/LConn2
  Steer/LConn4 -- Chassis/RConn3
  Steer/RConn4 -- Frame/LConn3
  Chassis/RConn5 -- Simscape Bus/LConn1
  Simscape Bus/LConn2 -- Chassis/RConn4
  Dtr/RConn1 -- Simscape Bus/RConn1
  Steer/LConn1 -- Connection Label/LConn1
  Connection Label1/LConn1 -- Steer/RConn1
  Act/RConn1 -- Simscape Bus1/RConn1
  Connection Label4/LConn1 -- Implement/RConn1
  Connection Label5/LConn1 -- Implement/RConn2
  Connection Label8/LConn1 -- Implement/RConn3
  Connection Label2/LConn1 -- Simscape Bus1/LConn1
  Simscape Bus1/LConn2 -- Connection Label3/LConn1
  Connection Label6/LConn1 -- Simscape Bus1/LConn3
  Connection Label7/LConn1 -- Simscape Bus1/LConn4
  Connection Label9/LConn1 -- Simscape Bus1/LConn5
  Camera Frames F/LConn1 -- Frame/RConn5 -- RefF/RConn1
  Camera Frames R/LConn1 -- Chassis/LConn1 -- RefR/RConn1

== system sm_mining_loader_lib/Mining Loader/Actuation/Lift ==
  Cmd : Inport
  Meas : Inport  Port=2
  Position : Subsystem  VariantControl=Position
      mask Display: image('sm_mining_loader_actuation_Position_IMAGE.png')
  Shaft : $bdroot/Shaft 2  VariantControl=Shaft  Kp=minMachParams.Control.Lift.propGain  Ki=minMachParams.Control.Lift.intgGain  Kd=minMachParams.Control.Lift.dervGain  p_init=minMachParams.Control.Lift.initPos  popup_act_pair=Parallel
  L : PMIOPort  Side=Right
  R : PMIOPort  Port=2  Side=Right

== system sm_mining_loader_lib/Mining Loader/Actuation/Steer ==
  Cmd : Inport
  Meas : Inport  Port=2
  Position : Subsystem  VariantControl=Position
      mask Display: image('sm_mining_loader_actuation_Position_IMAGE.png')
  Shaft : $bdroot/Shaft 2  VariantControl=Shaft  Kp=minMachParams.Control.Steer.propGain  Ki=minMachParams.Control.Steer.intgGain  Kd=minMachParams.Control.Steer.dervGain  p_init=minMachParams.Control.Steer.initPos  popup_act_pair=Opposing
  L : PMIOPort  Side=Right
  R : PMIOPort  Port=2  Side=Right

== system sm_mining_loader_lib/Mining Loader/Actuation/Tilt ==
  Cmd : Inport
  Meas : Inport  Port=2
  Position : Subsystem  VariantControl=Position
      mask Display: image('sm_mining_loader_actuation_Position_IMAGE.png')
  Shaft : $bdroot/Shaft  VariantControl=Shaft  Kp=minMachParams.Control.Tilt.propGain  Ki=minMachParams.Control.Tilt.intgGain  Kd=minMachParams.Control.Tilt.dervGain  p_init=minMachParams.Control.Tilt.initPos  f_init=-4.07e4*3
  R : PMIOPort  Side=Right

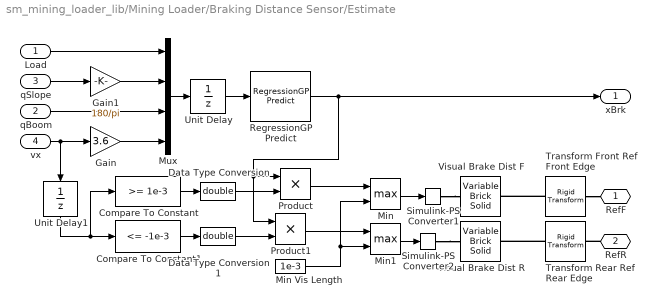
== system sm_mining_loader_lib/Mining Loader/Braking Distance Sensor/Estimate ==
  Load : Inport
  qBoom : Inport  Port=2
  qSlope : Inport  Port=3
  vx : Inport  Port=4
  Compare To Constant : simulink/Logic and Bit Operations/Compare To Constant  relop=>=  const=1e-3  OutDataTypeStr=uint8  ZeroCross=off
  Compare To Constant1 : simulink/Logic and Bit Operations/Compare To Constant  relop=<=  const=-1e-3  OutDataTypeStr=uint8  ZeroCross=off
  Data Type Conversion : DataTypeConversion  OutDataTypeStr=double  SaturateOnIntegerOverflow=off  RndMeth=Floor
  Data Type Conversion1 : DataTypeConversion  OutDataTypeStr=double  SaturateOnIntegerOverflow=off  RndMeth=Floor
  Gain : Gain  Gain=3.6
  Gain1 : Gain  Gain=180/pi
  Min : MinMax  Function=max  Inputs=2  ZeroCross=off
  Min Vis Length : Constant  Value=1e-3
  Min1 : MinMax  Function=max  Inputs=2  ZeroCross=off
  Mux : Mux
  Product : Product
  Product1 : Product
  RegressionGP Predict : statsLibrary/Regression/RegressionGP Predict  TrainedLearner=gpMdlCompact  ShowOutputSD=off  ShowOutputIntervals=off  Alpha=0.05  OutMin=[]  OutMax=[]  SDOutMin=[]  SDOutMax=[]  IntervalsOutMin=[]  IntervalsOutMax=[]  KernelMin=[]  KernelMax=[]  DistanceOutMin=[]  DistanceOutMax=[]  BasisOutMin=[]  BasisOutMax=[]  StandardizedInputOutMin=[]  StandardizedInputOutMax=[]  KernelParam1Min=[]  KernelParam1Max=[]  KernelParam2Min=[]  KernelParam2Max=[]  KernelParam3Min=[]  KernelParam3Max=[]  KernelParam4Min=[]  KernelParam4Max=[]  BasisParam1Min=[]  BasisParam1Max=[]  BasisParam2Min=[]  BasisParam2Max=[]  SDParam1Min=[]  SDParam1Max=[]  KernelParam5Min=[]  KernelParam5Max=[]
  Simulink-PS Converter1 : nesl_utility/Simulink-PS Converter  PhysicalDomain=network_engine_domain  SubClassName=ps_input  LeftPortType=input  RightPortType=output  PseudoPeriodic=off  Frequencies=[]  NoiseDistribution=none  NoiseParameters=[]  Unit=1  AffineConversion=off  FilteringAndDerivatives=provide  SimscapeFilterOrder=1  InputFilterTimeConstant=0.001  UdotUserProvided=0
  Simulink-PS Converter2 : nesl_utility/Simulink-PS Converter  PhysicalDomain=network_engine_domain  SubClassName=ps_input  LeftPortType=input  RightPortType=output  PseudoPeriodic=off  Frequencies=[]  NoiseDistribution=none  NoiseParameters=[]  Unit=1  AffineConversion=off  FilteringAndDerivatives=provide  SimscapeFilterOrder=1  InputFilterTimeConstant=0.001  UdotUserProvided=0
  Transform Front Ref Front Edge : sm_lib/Frames and Transforms/Rigid Transform  RotationMethod=StandardAxis  FollAlignAxisA=+X  BaseAlignAxisA=+Y  FollAlignAxisB=+Y  BaseAlignAxisB=+Z  RotationStandardAxis=+Y  RotationAngle=90  RotationAngleUnits=deg  RotationArbitraryAxis=[0 0 1]  RotationSequenceAxes=FollowerAxes  RotationSequence=XYX  RotationSequenceAngles=[0 0 0]  RotationSequenceAnglesUnits=deg  RotationMatrix=[1 0 0;0 1 0;0 0 1]  Quaternion=[1 0 0 0]  TranslationMethod=Cartesian  TranslationCartesianOffset=minMachParams.visual.frameRefToBucketEdge  TranslationCartesianOffsetUnits=m  TranslationStandardAxis=+X  TranslationStandardOffset=4.15  TranslationStandardOffsetUnits=m  TranslationROffset=0  TranslationROffsetUnits=m  TranslationThetaOffset=0  TranslationThetaOffsetUnits=deg  TranslationZOffset=0  TranslationZOffsetUnits=m
  Transform Rear Ref Rear Edge : sm_lib/Frames and Transforms/Rigid Transform  RotationMethod=StandardAxis  FollAlignAxisA=+X  BaseAlignAxisA=+Y  FollAlignAxisB=+Y  BaseAlignAxisB=+Z  RotationStandardAxis=+Y  RotationAngle=-90  RotationAngleUnits=deg  RotationArbitraryAxis=[0 0 1]  RotationSequenceAxes=FollowerAxes  RotationSequence=XYX  RotationSequenceAngles=[0 0 0]  RotationSequenceAnglesUnits=deg  RotationMatrix=[1 0 0;0 1 0;0 0 1]  Quaternion=[1 0 0 0]  TranslationMethod=Cartesian  TranslationCartesianOffset=minMachParams.visual.chassisRefToRearEdge  TranslationCartesianOffsetUnits=m  TranslationStandardAxis=+X  TranslationStandardOffset=-3.125  TranslationStandardOffsetUnits=m  TranslationROffset=0  TranslationROffsetUnits=m  TranslationThetaOffset=0  TranslationThetaOffsetUnits=deg  TranslationZOffset=0  TranslationZOffsetUnits=m
  Unit Delay : UnitDelay  InitialCondition=[0 0 0 0]  SampleTime=TsVis
  Unit Delay1 : UnitDelay  SampleTime=TsVis
  Visual Brake Dist F : sm_lib/Body Elements/Variable Mass/Variable Brick Solid  ComputedVariable=Density  XLengthType=Constant  XLength=0.01  XLengthUnits=m  YLengthType=Constant  YLength=3  YLengthUnits=m  ZLengthType=ProvidedByInput  ZLength=0.05  ZLengthUnits=m  DensityType=Constant  Density=1000  DensityUnits=kg/m^3  MassType=Constant  Mass=0.03  MassUnits=kg  SenseXLength=off  SenseYLength=off  SenseZLength=off  SenseDensity=off  SenseMass=off  SenseCenterOfMass=off  SenseInertiaMatrix=off  GraphicType=FromGeometry  MarkerShape=Sphere  MarkerSize=10  GraphicVisPropType=SimpleVisualProperties  GraphicDiffuseColor=minMachParams.visual.clr  GraphicOpacity=minMachParams.visual.opc  GraphicSpecularColor=[0.5 0.5 0.5 1.0]  GraphicAmbientColor=[0.15 0.15 0.15 1.0]  GraphicEmissiveColor=[0.0 0.0 0.0 1.0]  GraphicShininess=75
  Visual Brake Dist R : sm_lib/Body Elements/Variable Mass/Variable Brick Solid  ComputedVariable=Density  XLengthType=Constant  XLength=0.01  XLengthUnits=m  YLengthType=Constant  YLength=3  YLengthUnits=m  ZLengthType=ProvidedByInput  ZLength=0.05  ZLengthUnits=m  DensityType=Constant  Density=1000  DensityUnits=kg/m^3  MassType=Constant  Mass=0.03  MassUnits=kg  SenseXLength=off  SenseYLength=off  SenseZLength=off  SenseDensity=off  SenseMass=off  SenseCenterOfMass=off  SenseInertiaMatrix=off  GraphicType=FromGeometry  MarkerShape=Sphere  MarkerSize=10  GraphicVisPropType=SimpleVisualProperties  GraphicDiffuseColor=minMachParams.visual.clr  GraphicOpacity=minMachParams.visual.opc  GraphicSpecularColor=[0.5 0.5 0.5 1.0]  GraphicAmbientColor=[0.15 0.15 0.15 1.0]  GraphicEmissiveColor=[0.0 0.0 0.0 1.0]  GraphicShininess=75
  RefF : PMIOPort  Side=Right
  RefR : PMIOPort  Port=2  Side=Right
  xBrk : Outport
  wires:
  Unit Delay1/1 -> Compare To Constant1/1, Compare To Constant/1
  Product1/1 -> Min1/1
  Product/1 -> Min/1
  Gain1/1 -> Mux/2
  Unit Delay/1 -> RegressionGP Predict/1
  Mux/1 -> Unit Delay/1
  vx/1 -> Unit Delay1/1, Gain/1
  qSlope/1 -> Gain1/1
  Load/1 -> Mux/1
  qBoom/1 -> Mux/3
  Gain/1 -> Mux/4
  Compare To Constant/1 -> Data Type Conversion/1
  RegressionGP Predict/1 -> xBrk/1, Product1/1, Product/1
  Compare To Constant1/1 -> Data Type Conversion1/1
  Min/1 -> Simulink-PS Converter1/1
  Min Vis Length/1 -> Min1/2, Min/2
  Min1/1 -> Simulink-PS Converter2/1
  Data Type Conversion/1 -> Product/2
  Data Type Conversion1/1 -> Product1/2
  connections:
  Transform Front Ref Front Edge/LConn1 -- RefF/RConn1
  Transform Front Ref Front Edge/RConn1 -- Visual Brake Dist F/RConn1
  Simulink-PS Converter1/RConn1 -- Visual Brake Dist F/LConn1
  Transform Rear Ref Rear Edge/RConn1 -- Visual Brake Dist R/RConn1
  Simulink-PS Converter2/RConn1 -- Visual Brake Dist R/LConn1
  RefR/RConn1 -- Transform Rear Ref Rear Edge/LConn1

== system sm_mining_loader_lib/Mining Loader/Braking Distance Sensor/None ==
  Load : Inport
  qBoom : Inport  Port=2
  qSlope : Inport  Port=3
  vx : Inport  Port=4
  Constant : Constant  Value=0
  Reference Frame : sm_lib/Frames and Transforms/Reference Frame
  Reference Frame1 : sm_lib/Frames and Transforms/Reference Frame
  Terminator{,1..3} (4 alike) : Terminator
  RefF : PMIOPort  Side=Right
  RefR : PMIOPort  Port=2  Side=Right
  xBrk : Outport
  wires:
  Constant/1 -> xBrk/1
  qBoom/1 -> Terminator2/1
  Load/1 -> Terminator/1
  qSlope/1 -> Terminator1/1
  vx/1 -> Terminator3/1
  connections:
  RefF/RConn1 -- Reference Frame/RConn1
  Reference Frame1/RConn1 -- RefR/RConn1

== system sm_mining_loader_lib/Mining Loader/Scene/Grid ==
  Constant : Constant  Value=0
  Grid : grid_element/Grid  VariantControl=Grid  grid_x=SceneData.Grid.len  grid_y=SceneData.Grid.wid  grid_z=SceneData.Grid.dep  grid_line_width=SceneData.Grid.line_wid  grid_num_sq_x=SceneData.Grid.nsq_x  grid_num_sq_y=SceneData.Grid.nsq_y  grid_clr=SceneData.Grid.line_clr  plane_clr=SceneData.Grid.surf_clr  grid_opc=SceneData.Grid.line_opc  plane_opc=SceneData.Grid.surf_opc
  Infinite Plane : sm_lib/Curves and Surfaces/Infinite Plane  GraphicType=Rectangle  GraphicPlaneWidth=1  GraphicPlaneWidthUnits=m  GraphicPlaneHeight=1  GraphicPlaneHeightUnits=m  GraphicVisPropType=SimpleVisualProperties  GraphicDiffuseColor=[0.5 0.5 0.5]  GraphicOpacity=1  GraphicSpecularColor=[0.5 0.5 0.5 1.0]  GraphicAmbientColor=[0.15 0.15 0.15 1.0]  GraphicEmissiveColor=[0.0 0.0 0.0 1.0]  GraphicShininess=75
  Path : sm_lib/Curves and Surfaces/Spline  DataPoints=[Maneuver.Trajectory.x.Value' Maneuver.Trajectory.y.Value' Maneuver.Trajectory.z.Value']  DataPointsUnits=m  EndConditionType=Natural  GraphicType=FromGeometry  MarkerShape=Sphere  MarkerSize=10  GraphicVisPropType=SimpleVisualProperties  GraphicDiffuseColor=[0 0 0]  GraphicOpacity=1  GraphicSpecularColor=[0.5 0.5 0.5 1.0]  GraphicAmbientColor=[0.15 0.15 0.15 1.0]  GraphicEmissiveColor=[0.0 0.0 0.0 1.0]  GraphicShininess=75
  G : PMIOPort  Side=Right
  W : PMIOPort  Port=2  Side=Left
  Out Bus Element : Outport  PortName=m  Element=Slope
  wires:
  Constant/1 -> Out Bus Element/1  "Slope"
  connections:
  Grid/RConn1 -- W/RConn1 -- Path/LConn1 -- Infinite Plane/LConn1
  Infinite Plane/RConn1 -- G/RConn1

== system sm_mining_loader_lib/Mining Loader/Scene/SlopeX ==
  Infinite Plane : sm_lib/Curves and Surfaces/Infinite Plane  GraphicType=Rectangle  GraphicPlaneWidth=60  GraphicPlaneWidthUnits=m  GraphicPlaneHeight=4  GraphicPlaneHeightUnits=m  GraphicVisPropType=SimpleVisualProperties  GraphicDiffuseColor=[0.5 0.5 0.5]  GraphicOpacity=0.5  GraphicSpecularColor=[0.5 0.5 0.5 1.0]  GraphicAmbientColor=[0.15 0.15 0.15 1.0]  GraphicEmissiveColor=[0.0 0.0 0.0 1.0]  GraphicShininess=75
  Slope : Constant  Value=Init.Vehicle.pitch
  Transform Slope : sm_lib/Frames and Transforms/Rigid Transform  RotationMethod=StandardAxis  FollAlignAxisA=+X  BaseAlignAxisA=+Y  FollAlignAxisB=+Y  BaseAlignAxisB=+Z  RotationStandardAxis=+Y  RotationAngle=Init.Vehicle.pitch  RotationAngleUnits=deg  RotationArbitraryAxis=[0 0 1]  RotationSequenceAxes=BaseAxes  RotationSequence=XYZ  RotationSequenceAngles=[0 0 0]  RotationSequenceAnglesUnits=deg  RotationMatrix=[1 0 0;0 1 0;0 0 1]  Quaternion=[1 0 0 0]  TranslationMethod=None  TranslationCartesianOffset=[0 0 0]  TranslationCartesianOffsetUnits=m  TranslationStandardAxis=+Z  TranslationStandardOffset=0  TranslationStandardOffsetUnits=m  TranslationROffset=0  TranslationROffsetUnits=m  TranslationThetaOffset=0  TranslationThetaOffsetUnits=deg  TranslationZOffset=0  TranslationZOffsetUnits=m
  G : PMIOPort  Side=Right
  W : PMIOPort  Port=2  Side=Left
  Out Bus Element : Outport  PortName=m  Element=Slope
  wires:
  Slope/1 -> Out Bus Element/1  "Slope"
  connections:
  Infinite Plane/RConn1 -- G/RConn1
  Transform Slope/RConn1 -- Infinite Plane/LConn1
  Transform Slope/LConn1 -- W/RConn1
